simulink model "simscape_language_validation"  (R2024a)
settings: Solver=VariableStepAuto  StartTime=0.0  StopTime=30*60  RelTol=1e-3
libraries: fl_lib x16, nesl_utility x10
settings Model: Creator=jvansick  LastModifiedBy=jvansick

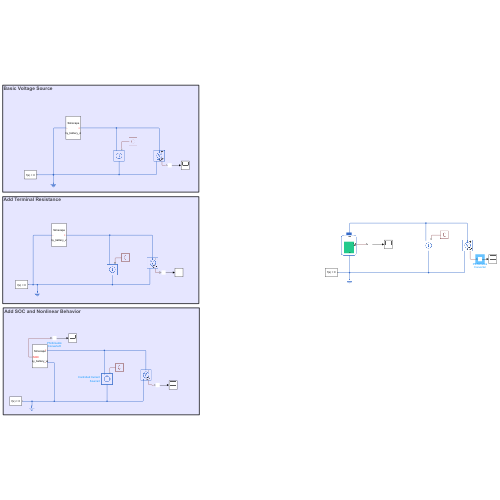
[thumbnail: Simulink's stored preview of the top-level diagram]
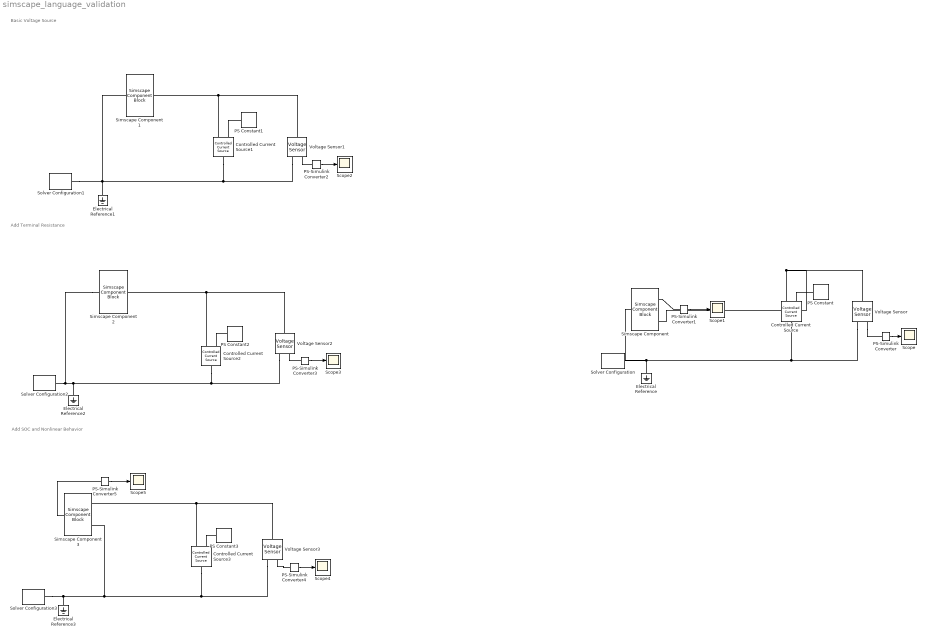
== system simscape_language_validation ==
  note: Add SOC and Nonlinear Behavior
  note: Basic Voltage Source
  note: Add Terminal Resistance
  Controlled Current Source{,1..3} (4 alike) : fl_lib/Electrical/Electrical Sources/Controlled Current Source
  Electrical Reference{,1..3} (4 alike) : fl_lib/Electrical/Electrical Elements/Electrical Reference
  PS Constant{,1..3} (4 alike) : fl_lib/Physical Signals/Sources/PS Constant  constant=10 A
  PS-Simulink Converter{,1..5} (6 alike) : nesl_utility/PS-Simulink Converter  PhysicalDomain=network_engine_domain  SubClassName=ps_output  LeftPortType=input  RightPortType=output  PseudoPeriodic=off  Frequencies=[]  VectorFormat=inherit  Unit=inherit  AffineConversion=off
  Scope{,1..5} (6 alike) : Scope
  Simscape Component : SimscapeComponentBlock  SourceFile=my_battery  ComponentPath=my_battery  ComponentVariants="[\"my_battery\"]"  ComponentVariantNames="[\"my_battery\"]"  ClassName=my_battery  SchemaVersion=1  nominal_voltage=10 V  AH_rating=5 A*hr  terminal_resistance=0.02 Ohm  voltage_data=[0, 1, 9, 10, 11] V  SOC_data=[0, .05, .2, .95, 1]  i_specify=off  i_priority=None  i=0 A  i_nominal_specify=off  i_nominal_value=1  i_nominal_unit=A  v_specify=off  v_priority=None  v=0 V  v_nominal_specify=off  v_nominal_value=1  v_nominal_unit=V  SOC_specify=on  SOC_priority=High  SOC=1  SOC_nominal_specify=off  SOC_nominal_value=1  SOC_nominal_unit=1
      settings: CopyFcn=simscape.engine.sli.internal.componentblockcallback(gcbh,'COPY')  PreCopyFcn=simscape.engine.sli.internal.componentblockcallback(gcbh,'PRECOPY')  PreDeleteFcn=simscape.engine.sli.internal.componentblockcallback(gcbh,'PREDELETE')  InternalSimscapePortConfiguration="{\"Bottom\":[{\"id\":\"n\",\"label\":\"-\",\"type\":\"foundation.electrical.electrical\"}],\"Left\":[{\"id\":\"SOC_out\",\"label\":\"S\",\"type\":\"output\"}],\"Right\":[],\"Top\":[{\"id\":\"p\",\"label\":\"+\",\"type\":\"foundation.electrical.electrical\"}]}"
      mask Type: My Battery
  Simscape Component1 : SimscapeComponentBlock  SourceFile=my_battery_v0  ComponentPath=my_battery_v0  ComponentVariants="[\"my_battery_v0\"]"  ComponentVariantNames="[\"my_battery_v0\"]"  ClassName=my_battery_v0  SchemaVersion=1  nominal_voltage=10 V  i_specify=off  i_priority=None  i=0 A  i_nominal_specify=off  i_nominal_value=1  i_nominal_unit=A  v_specify=off  v_priority=None  v=0 V  v_nominal_specify=off  v_nominal_value=1  v_nominal_unit=V
      settings: CopyFcn=simscape.engine.sli.internal.componentblockcallback(gcbh,'COPY')  PreCopyFcn=simscape.engine.sli.internal.componentblockcallback(gcbh,'PRECOPY')  PreDeleteFcn=simscape.engine.sli.internal.componentblockcallback(gcbh,'PREDELETE')  InternalSimscapePortConfiguration="{\"Bottom\":[],\"Left\":[{\"id\":\"p\",\"label\":\"+\",\"type\":\"foundation.electrical.electrical\"}],\"Right\":[{\"id\":\"n\",\"label\":\"-\",\"type\":\"foundation.electrical.electrical\"}],\"Top\":[]}"
      mask Type: My Battery
  Simscape Component2 : SimscapeComponentBlock  SourceFile=my_battery_v1  ComponentPath=my_battery_v1  ComponentVariants="[\"my_battery_v1\"]"  ComponentVariantNames="[\"my_battery_v1\"]"  ClassName=my_battery_v1  SchemaVersion=1  nominal_voltage=10 V  terminal_resistance=0.02 Ohm  i_specify=off  i_priority=None  i=0 A  i_nominal_specify=off  i_nominal_value=1  i_nominal_unit=A  v_specify=off  v_priority=None  v=0 V  v_nominal_specify=off  v_nominal_value=1  v_nominal_unit=V
      settings: CopyFcn=simscape.engine.sli.internal.componentblockcallback(gcbh,'COPY')  PreCopyFcn=simscape.engine.sli.internal.componentblockcallback(gcbh,'PRECOPY')  PreDeleteFcn=simscape.engine.sli.internal.componentblockcallback(gcbh,'PREDELETE')  InternalSimscapePortConfiguration="{\"Bottom\":[],\"Left\":[{\"id\":\"p\",\"label\":\"+\",\"type\":\"foundation.electrical.electrical\"}],\"Right\":[{\"id\":\"n\",\"label\":\"-\",\"type\":\"foundation.electrical.electrical\"}],\"Top\":[]}"
      mask Type: My Battery
  Simscape Component3 : SimscapeComponentBlock  SourceFile=my_battery_v2  ComponentPath=my_battery_v2  ComponentVariants="[\"my_battery_v2\"]"  ComponentVariantNames="[\"my_battery_v2\"]"  ClassName=my_battery_v2  SchemaVersion=1  nominal_voltage=10 V  AH_rating=5 A*hr  terminal_resistance=0.02 Ohm  voltage_data=[0, 1, 9, 10, 11] V  SOC_data=[0, .05, .2, .95, 1]  i_specify=off  i_priority=None  i=0 A  i_nominal_specify=off  i_nominal_value=1  i_nominal_unit=A  v_specify=off  v_priority=None  v=0 V  v_nominal_specify=off  v_nominal_value=1  v_nominal_unit=V  SOC_specify=off  SOC_priority=None  SOC=1  SOC_nominal_specify=off  SOC_nominal_value=1  SOC_nominal_unit=1
      settings: CopyFcn=simscape.engine.sli.internal.componentblockcallback(gcbh,'COPY')  PreCopyFcn=simscape.engine.sli.internal.componentblockcallback(gcbh,'PRECOPY')  PreDeleteFcn=simscape.engine.sli.internal.componentblockcallback(gcbh,'PREDELETE')  InternalSimscapePortConfiguration="{\"Bottom\":[],\"Left\":[{\"id\":\"p\",\"label\":\"+\",\"type\":\"foundation.electrical.electrical\"},{\"id\":\"n\",\"label\":\"-\",\"type\":\"foundation.electrical.electrical\"}],\"Right\":[{\"id\":\"SOC_out\",\"label\":\"SOC\",\"type\":\"output\"}],\"Top\":[]}"
      mask Type: My Battery
  Solver Configuration{,1..3} (4 alike) : nesl_utility/Solver Configuration  PhysicalDomain=network_engine_domain  SubClassName=solver  LeftPortType=input  RightPortType=generic  Tones=[]  Harmonics=[]  SimulateNoise=off  Profile=off  UseLocalSampling=off  EnableSwitchedLinearOptims=on  FrequencyDomain=off  UseCCode=off  RelTol=0.001  AbsTol=0.001  MinStep=1e-09  ToWorkspace=off  RevertToSquareIcSolve=off  NumHomotopyIterations=100  PhasorMode=off  PhasorModeNumHarmonics=1  ConsistencySolver=NEWTON_XTOL_AFTER_FTOL  IndexReductionMethod=DerivativeReplacement  DoDC=off  ResidualTolerance=1e-09  ConsistencyTolSource=GLOBAL  ConsistencyAbsTol=0.001  ConsistencyRelTol=0.001  ConsistencyTolFactor=0.001  UseLocalSolver=off  LocalSolverChoice=NE_BACKWARD_EULER_ADVANCER  ResolveIndetEquations=on  FunctionEvalNumThread=1  LocalSolverSampleTime=0.001  DoFixedCost=off  MaxNonlinIter=3  MaxModeIter=2  ComputeImpulses=off  ImpulseIterations=2  LinearAlgebra=auto  LinearAlgebraNumThread=0  EquationFormulation=NE_TIME_EF  DelaysMemoryBudget=1024  AutomaticFiltering=on  FilteringTimeConstant=0.001  PartitionStorageMethod=AS_NEEDED  PartitionMemoryBudget=1024  PartitionMethod=ROBUST  MultibodyUseLocalSolver=off  MultibodyLocalSolverChoice=ODE1  MultibodyLocalSolverSampleTime=0.001
  Voltage Sensor{,1..3} (4 alike) : fl_lib/Electrical/Electrical Sensors/Voltage Sensor
  wires:
  PS-Simulink Converter/1 -> Scope/1
  PS-Simulink Converter1/1 -> Scope1/1
  PS-Simulink Converter2/1 -> Scope2/1
  PS-Simulink Converter3/1 -> Scope3/1
  PS-Simulink Converter4/1 -> Scope4/1
  PS-Simulink Converter5/1 -> Scope5/1
  connections:
  Electrical Reference/LConn1 -- Voltage Sensor/RConn2 -- Controlled Current Source/LConn1 -- Solver Configuration/RConn1 -- Simscape Component/RConn1
  PS Constant/RConn1 -- Controlled Current Source/RConn1
  Voltage Sensor/RConn1 -- PS-Simulink Converter/LConn1
  PS-Simulink Converter1/LConn1 -- Simscape Component/LConn1
  Controlled Current Source/RConn2 -- Simscape Component/LConn2 -- Voltage Sensor/LConn1
  Electrical Reference1/LConn1 -- Voltage Sensor1/RConn2 -- Controlled Current Source1/LConn1 -- Simscape Component1/RConn1 -- Solver Configuration1/RConn1
  Controlled Current Source1/RConn2 -- Voltage Sensor1/LConn1 -- Simscape Component1/LConn1
  Voltage Sensor1/RConn1 -- PS-Simulink Converter2/LConn1
  PS Constant1/RConn1 -- Controlled Current Source1/RConn1
  Simscape Component2/RConn1 -- Electrical Reference2/LConn1 -- Voltage Sensor2/RConn2 -- Controlled Current Source2/LConn1 -- Solver Configuration2/RConn1
  Controlled Current Source2/RConn2 -- Simscape Component2/LConn1 -- Voltage Sensor2/LConn1
  PS Constant2/RConn1 -- Controlled Current Source2/RConn1
  Voltage Sensor2/RConn1 -- PS-Simulink Converter3/LConn1
  Voltage Sensor3/RConn2 -- Solver Configuration3/RConn1 -- Electrical Reference3/LConn1 -- Simscape Component3/LConn2 -- Controlled Current Source3/LConn1
  Simscape Component3/LConn1 -- Voltage Sensor3/LConn1 -- Controlled Current Source3/RConn2
  Voltage Sensor3/RConn1 -- PS-Simulink Converter4/LConn1
  PS Constant3/RConn1 -- Controlled Current Source3/RConn1
  PS-Simulink Converter5/LConn1 -- Simscape Component3/RConn1
